simulink model "abe_simulink_model_v2"  (R2022a)
settings: Solver=VariableStepAuto  StartTime=0  StopTime=50  RelTol=1e-3
libraries: simulink x1
settings Model: Creator=Abraham  LastModifiedBy=Abraham

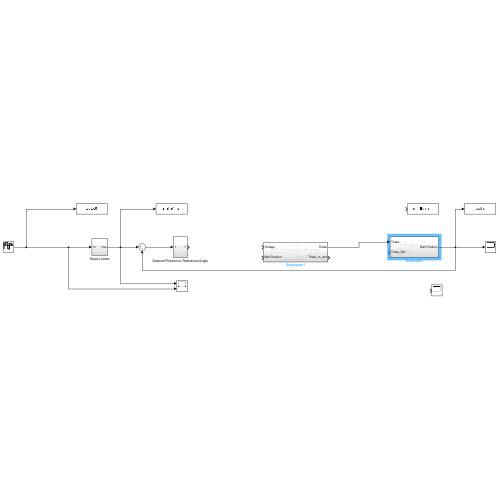
[thumbnail: Simulink's stored preview of the top-level diagram]
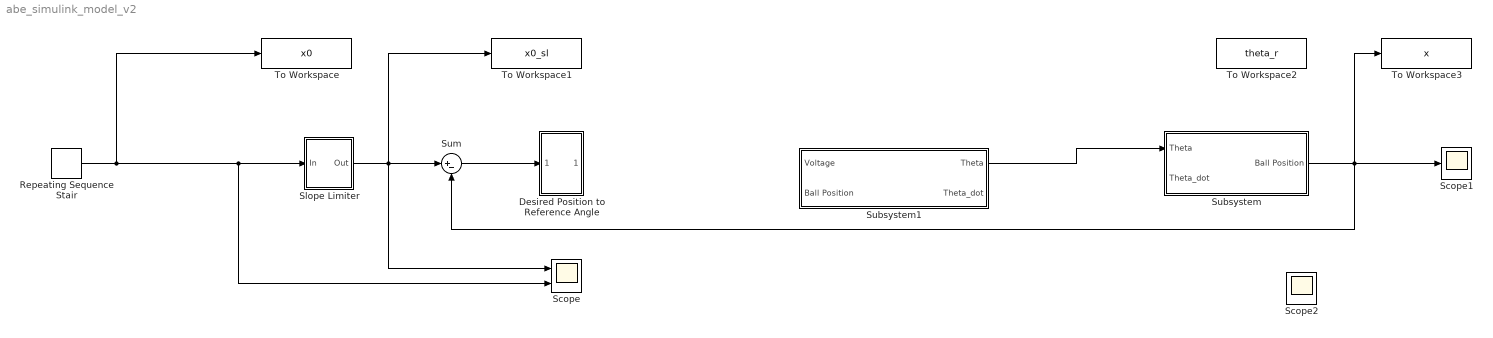
== system abe_simulink_model_v2 ==
  Desired Position to Reference Angle : Subsystem
  Repeating Sequence Stair : simulink/Sources/Repeating Sequence Stair  OutValues=[5 15 -20 10 0]  tsamp=10  OutMin=[]  OutMax=[]  OutDataTypeStr=double  OutputDataTypeScalingMode=double  OutDataType=fixdt(0,8)  ConRadixGroup=Best Precision: Vector-wise  OutScaling=2^-12
  Scope : Scope  NumInputPorts=2
  Scope1 : Scope
  Scope2 : Scope
  Slope Limiter : Subsystem
  Subsystem : Subsystem
  Subsystem1 : Subsystem
  Sum : Sum  Inputs=|+-
  To Workspace : ToWorkspace  VariableName=x0  SaveFormat=Timeseries  SampleTime=-1
  To Workspace1 : ToWorkspace  VariableName=x0_sl  SaveFormat=Timeseries  SampleTime=-1
  To Workspace2 : ToWorkspace  VariableName=theta_r  SaveFormat=Timeseries  SampleTime=-1
  To Workspace3 : ToWorkspace  VariableName=x  SaveFormat=Timeseries  SampleTime=-1
  wires:
  Slope Limiter/1(Out) -> Sum/1, To Workspace1/1, Scope/1
  Repeating Sequence Stair/1 -> To Workspace/1, Scope/2, Slope Limiter/1(In)
  Sum/1 -> Desired Position to Reference Angle/1(In1)
  Subsystem/1(Ball Position) -> Sum/2, To Workspace3/1, Scope1/1
  Subsystem1/1(Theta) -> Subsystem/1(Theta)

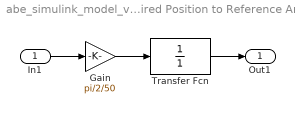
== system abe_simulink_model_v2/Desired Position to Reference Angle ==
  In1 : Inport
  Gain : Gain  Gain=pi/2/50
  Transfer Fcn : TransferFcn  Denominator=[1]
  Out1 : Outport
  wires:
  Gain/1 -> Transfer Fcn/1
  In1/1 -> Gain/1
  Transfer Fcn/1 -> Out1/1

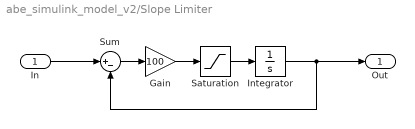
== system abe_simulink_model_v2/Slope Limiter ==
  In : Inport
  Gain : Gain  Gain=100
  Integrator : Integrator
  Saturation : Saturate  UpperLimit=10  LowerLimit=-10
  Sum : Sum  Inputs=|+-
  Out : Outport
  wires:
  Integrator/1 -> Out/1, Sum/2
  Gain/1 -> Saturation/1
  Saturation/1 -> Integrator/1
  Sum/1 -> Gain/1
  In/1 -> Sum/1

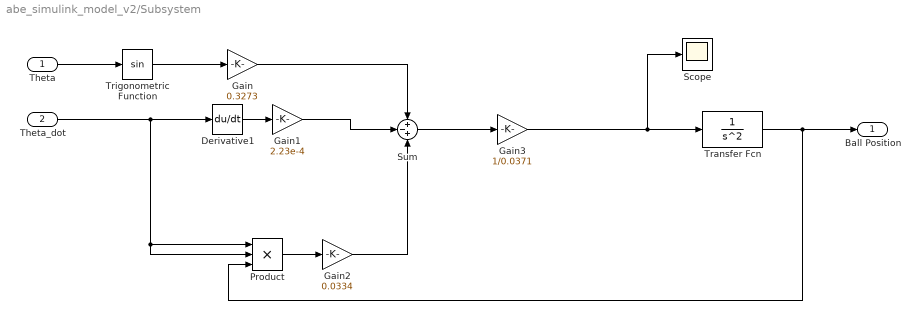
== system abe_simulink_model_v2/Subsystem ==
  Theta : Inport
  Theta_dot : Inport  Port=2
  Derivative1 : Derivative
  Gain : Gain  Gain=0.3273
  Gain1 : Gain  Gain=2.23e-4
  Gain2 : Gain  Gain=0.0334
  Gain3 : Gain  Gain=1/0.0371
  Product : Product  Inputs=3
  Scope : Scope
  Sum : Sum  Inputs=+-+
  Transfer Fcn : TransferFcn  Denominator=[1 0 0]
  Trigonometric Function : Trigonometry
  Ball Position : Outport
  wires:
  Theta/1 -> Trigonometric Function/1
  Trigonometric Function/1 -> Gain/1
  Derivative1/1 -> Gain1/1
  Product/1 -> Gain2/1
  Transfer Fcn/1 -> Product/3, Ball Position/1
  Gain/1 -> Sum/1
  Gain1/1 -> Sum/2
  Gain2/1 -> Sum/3
  Sum/1 -> Gain3/1
  Gain3/1 -> Scope/1, Transfer Fcn/1
  Theta_dot/1 -> Product/2, Product/1, Derivative1/1

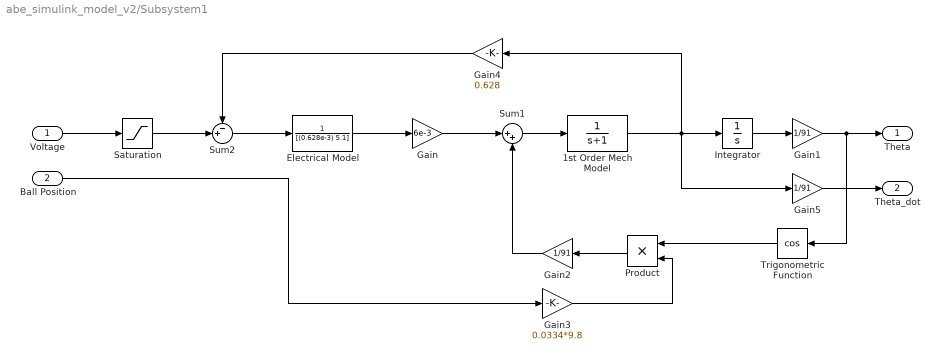
== system abe_simulink_model_v2/Subsystem1 ==
  Voltage : Inport
  Ball Position : Inport  Port=2
  1st Order Mech Model : TransferFcn  Denominator=[1 1]
  Electrical Model : TransferFcn  Denominator=[(0.628e-3) 5.1]
  Gain : Gain  Gain=6e-3
  Gain1 : Gain  Gain=1/91
  Gain2 : Gain  Gain=1/91
  Gain3 : Gain  Gain=0.0334*9.8
  Gain4 : Gain  Gain=0.628
  Gain5 : Gain  Gain=1/91
  Integrator : Integrator
  Product : Product
  Saturation : Saturate  UpperLimit=6  LowerLimit=-6
  Sum1 : Sum  Inputs=|++
  Sum2 : Sum  Inputs=-+|
  Trigonometric Function : Trigonometry  Operator=cos
  Theta : Outport
  Theta_dot : Outport  Port=2
  wires:
  Trigonometric Function/1 -> Product/1
  Sum2/1 -> Electrical Model/1
  Gain2/1 -> Sum1/2
  Gain3/1 -> Product/2
  Gain4/1 -> Sum2/1
  Saturation/1 -> Sum2/2
  Gain/1 -> Sum1/1
  Gain1/1 -> Theta/1, Trigonometric Function/1
  Electrical Model/1 -> Gain/1
  Product/1 -> Gain2/1
  Integrator/1 -> Gain1/1
  Sum1/1 -> 1st Order Mech Model/1
  Voltage/1 -> Saturation/1
  Ball Position/1 -> Gain3/1
  1st Order Mech Model/1 -> Gain4/1, Gain5/1, Integrator/1
  Gain5/1 -> Theta_dot/1
